simulink model "oven_model"  (R2026a)
settings: Solver=ode15s  StopTime=3600
values from neighbouring files (symbols this model uses):
  A_chimney = pi * D_chimney^2 / 4    (= 0.00785398163397)    [oven_parameters.m]    (also in oven_parameters_V1.m)
  A_floor = W_floor * L_floor    (= 0.3239)    [oven_parameters.m]    (also in oven_parameters_V1.m)
  A_pizza = pi * D_pizza^2 / 4    (= 0.0804247719319)    [oven_parameters.m]    (also in oven_parameters_V1.m)
  A_rad_roof_floor = A_floor    (= 0.3239)    [oven_parameters.m]    (also in oven_parameters_V1.m)
  A_rad_roof_pizza = A_pizza    (= 0.0804247719319)    [oven_parameters.m]    (also in oven_parameters_V1.m)
  A_roof = A_floor    (= 0.3239)    [oven_parameters.m]    (also in oven_parameters_V1.m)
  C_floor = m_floor * cp_floor    (= 7579.26)    [oven_parameters.m]    (also in oven_parameters_V1.m)
  C_gas = m_gas * cp_gas    (= 136.917)    [oven_parameters.m]    (also in oven_parameters_V1.m)
  C_pizza = m_pizza * cp_pizza    (= 625)    [oven_parameters.m]    (also in oven_parameters_V1.m)
  C_roof = m_roof * cp_roof    (= 2526.42)    [oven_parameters.m]    (also in oven_parameters_V1.m)
  Cd_chimney = 0.65    [oven_parameters.m]    (also in oven_parameters_V1.m)
  cp_gas = 1100    [oven_parameters.m]    (also in oven_parameters_V1.m)
  epsilon_pizza = 0.9    [oven_parameters.m]    (also in oven_parameters_V1.m)
  epsilon_roof = 0.8    [oven_parameters.m]    (also in oven_parameters_V1.m)
  g = oven_geometry(p)    [build_oven_simulink.m]    (also in oven_parameters.m = 9.81; oven_parameters_V1.m = 9.81; oven_refresh_model.m; run_oven_study.m = s.results{1}.g)
  H_chimney = 0.50    (= 0.5)    [oven_parameters.m]    (also in oven_parameters_V1.m)
  h_floor_pizza = 150    [oven_parameters.m]    (also in oven_parameters_V1.m)
  h_gas_floor = 20    [oven_parameters.m]    (also in oven_parameters_V1.m)
  h_gas_pizza = 10    [oven_parameters.m]    (also in oven_parameters_V1.m)
  h_gas_roof = 15    [oven_parameters.m]    (also in oven_parameters_V1.m)
  k_evap = 1e-5    (= 1e-05)    [oven_parameters.m]    (also in oven_parameters_V1.m)
  K_floor = 8    [oven_parameters.m]    (also in oven_parameters_V1.m)
  K_roof = 5    [oven_parameters.m]    (also in oven_parameters_V1.m)
  L_vap = 2.26e6    (= 2260000)    [oven_parameters.m]    (also in oven_parameters_V1.m)
  m_water_0 = water_fraction * m_pizza    (= 0.15)    [oven_parameters.m]    (also in oven_parameters_V1.m)
  P_ambient = 101325    [oven_parameters.m]    (also in oven_parameters_V1.m)
  Q_comb = mdot_wood * LHV_wood * eta_comb    (= 13755)    [oven_parameters.m]    (also in oven_parameters_V1.m = 5250)
  R_air = 287    [oven_parameters.m]    (also in oven_parameters_V1.m)
  rho_ambient = P_ambient / (R_air * T_ambient)    (= 1.184131412)    [oven_parameters.m]    (also in oven_parameters_V1.m)
  sigma = 5.670374419e-8    (= 5.670374419e-08)    [oven_parameters.m]    (also in oven_parameters_V1.m)
  T_ambient = 25 + 273.15    (= 298.15)    [oven_parameters.m]    (also in oven_parameters_V1.m)
  T_evap = 373.15    [oven_parameters.m]    (also in oven_parameters_V1.m)
  T_floor_0 = T_ambient    (= 298.15)    [oven_parameters.m]    (also in oven_parameters_V1.m)
  T_gas_0 = T_ambient    (= 298.15)    [oven_parameters.m]    (also in oven_parameters_V1.m)
  T_pizza_0 = T_ambient    (= 298.15)    [oven_parameters.m]    (also in oven_parameters_V1.m)
  T_roof_0 = T_ambient    (= 298.15)    [oven_parameters.m]    (also in oven_parameters_V1.m)
settings Model: Creator=samue  LastModifiedBy=samue

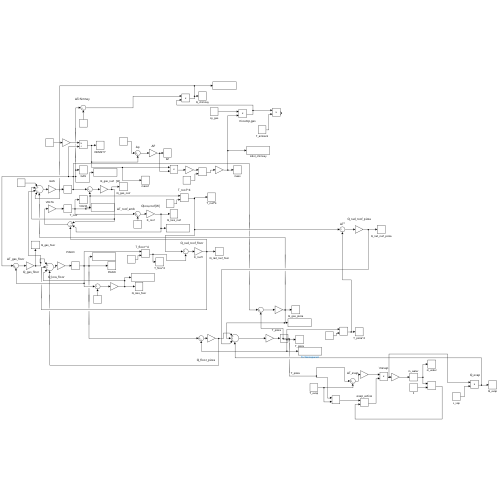
[thumbnail: Simulink's stored preview of the top-level diagram]
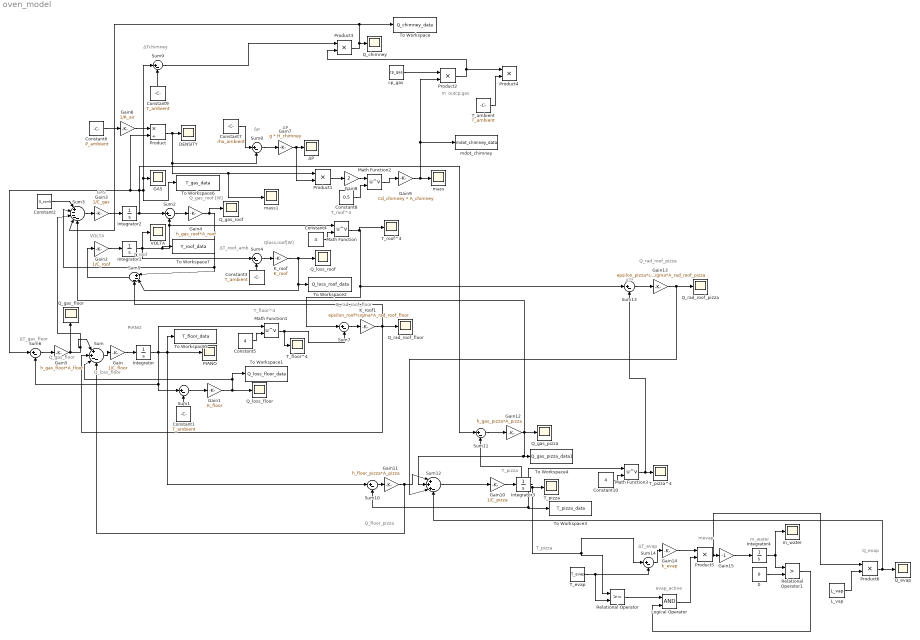
== system oven_model ==
  note: Q_evap
  note: evap_active
  note: ˙mevap​
  note: ΔT_evap
  note: T_pizza
  note: m_water
  note: Q_rad_roof_pizza
  note: ΔT⁴
  note: Q_floor_pizza
  note: T_pizza
  note: ΔTchimney​
  note: m˙out​cp,gas​
  note: ΔP
  note: Δρ
  note: Q_rad_roof_floor
  note: Q_loss_floor
  note: Q_gas_floor
  note: T_floor^4
  note: T_roof^4
  note: ΔT_gas_floor
  note: Qloss,roof​[W]
  note: ΔT_roof_amb
  note: T_roof
  note: Q_gas_roof [W]
  note: GAS
  note: VOLTA
  note: PIANO
  0 : Constant  Value=0
  Constant1 : Constant  Value=T_ambient
  Constant10 : Constant  Value=4
  Constant2 : Constant  Value=Q_comb
  Constant3 : Constant  Value=T_ambient
  Constant4 : Constant  Value=4
  Constant5 : Constant  Value=4
  Constant6 : Constant  Value=P_ambient
  Constant7 : Constant  Value=rho_ambient
  Constant8 : Constant  Value=0.5
  Constant9 : Constant  Value=T_ambient
  DENSITY : Scope
      settings: ActiveDisplayYMinimum=-0.56030182156001862  ActiveDisplayYMaximum=1.4111972218569013  DataLoggingVariableName=ScopeData3
  GAS : Scope
      settings: ActiveDisplayYMinimum=258.3429659927196  ActiveDisplayYMaximum=656.41330606552378
  Gain : Gain  Gain=1/C_floor
  Gain1 : Gain  Gain=K_floor
  Gain10 : Gain  Gain=1/C_pizza
  Gain11 : Gain  Gain=h_floor_pizza*A_pizza
  Gain12 : Gain  Gain=h_gas_pizza*A_pizza
  Gain13 : Gain  Gain=epsilon_pizza*sigma*A_rad_roof_pizza
  Gain14 : Gain  Gain=k_evap
  Gain15 : Gain  Gain=-1
  Gain2 : Gain  Gain=1/C_roof
  Gain3 : Gain  Gain=1/C_gas
  Gain4 : Gain  Gain=h_gas_roof*A_roof
  Gain5 : Gain  Gain=h_gas_floor*A_floor
  Gain6 : Gain  Gain=1/R_air
  Gain7 : Gain  Gain=g * H_chimney
  Gain8 : Gain  Gain=2
  Gain9 : Gain  Gain=Cd_chimney * A_chimney
  Integrator : Integrator  InitialCondition=T_floor_0
  Integrator1 : Integrator  InitialCondition=T_roof_0
  Integrator2 : Integrator  InitialCondition=T_gas_0
  Integrator3 : Integrator  InitialCondition=T_pizza_0
  Integrator4 : Integrator  InitialCondition=m_water_0
  K_roof : Gain  Gain=K_roof
  K_roof1 : Gain  Gain=epsilon_roof*sigma*A_rad_roof_floor
  L_vap : Constant  Value=L_vap
  Logical Operator : Logic  AllPortsSameDT=off  OutDataTypeStr=boolean
  Math Function{,1..3} (4 alike) : Math  Operator=pow
  PIANO : Scope
      settings: ActiveDisplayYMinimum=235.4778080469699  ActiveDisplayYMaximum=862.19972757727112
  Product : Product  Inputs=*/
  Product{1..4} (4 alike) : Product  Inputs=**
  Product5 : Product
  Product6 : Product
  Q_chimney : Scope
      settings: ActiveDisplayYMinimum=-981.18771548625477  ActiveDisplayYMaximum=8830.6894393762959  DataLoggingVariableName=Q_chimney_data
  Q_evap : Scope
      settings: ActiveDisplayYMinimum=-1268.2904261134306  ActiveDisplayYMaximum=11414.613835020878  DataLoggingVariableName=ScopeData20
  Q_gas_floor : Scope
      settings: ActiveDisplayYMinimum=-568.21387781314047  ActiveDisplayYMaximum=5113.9249003182649  DataLoggingVariableName=ScopeData9
  Q_gas_pizza : Scope
      settings: ActiveDisplayYMinimum=-24.642470577879937  ActiveDisplayYMaximum=221.7822352009195  DataLoggingVariableName=ScopeData16
  Q_gas_roof : Scope
      settings: ActiveDisplayYMinimum=-143.66606417495345  ActiveDisplayYMaximum=1292.9945775745814  DataLoggingVariableName=ScopeData10
  Q_loss_floor : Scope
      settings: ActiveDisplayYMinimum=-501.37753562424086  ActiveDisplayYMaximum=4512.3978206181691  DataLoggingVariableName=ScopeData11
  Q_loss_roof : Scope
      settings: ActiveDisplayYMinimum=-316.41135252661337  ActiveDisplayYMaximum=2847.7021727395208  DataLoggingVariableName=ScopeData15
  Q_rad_roof_floor : Scope
      settings: ActiveDisplayYMinimum=-13.468128699934045  ActiveDisplayYMaximum=121.21315829940644  DataLoggingVariableName=ScopeData12
  Q_rad_roof_pizza : Scope
      settings: ActiveDisplayYMinimum=-15.029157613821152  ActiveDisplayYMaximum=25.426795565679427  DataLoggingVariableName=ScopeData18
  Relational Operator : RelationalOperator  OutDataTypeStr=boolean  RndMeth=Simplest  InputSameDT=off
  Relational Operator1 : RelationalOperator  Operator=>  OutDataTypeStr=boolean  RndMeth=Simplest  InputSameDT=off
  Sum : Sum  Inputs=|++--
  Sum{1..2,4,6..11,13..14} (11 alike) : Sum  Inputs=|+-
  Sum12 : Sum  Inputs=|+++-
  Sum3 : Sum  Inputs=|+----
  Sum5 : Sum  Inputs=|+--
  T_ambient : Constant  Value=T_ambient
  T_evap : Constant  Value=T_evap
  T_floor^4 : Scope
      settings: ActiveDisplayYMinimum=-4.2189360590233528E+10  ActiveDisplayYMaximum=4.5872465094973682E+11  DataLoggingVariableName=ScopeData14
  T_pizza : Scope
      settings: ActiveDisplayYMinimum=232.78079290987318  ActiveDisplayYMaximum=886.47286381114156  DataLoggingVariableName=ScopeData7
  T_pizza^4 : Scope
      settings: ActiveDisplayYMinimum=3.7007260322625837E+9  ActiveDisplayYMaximum=4.57138713472718E+10  DataLoggingVariableName=ScopeData17
  T_roof^4 : Scope
      settings: ActiveDisplayYMinimum=-4.3448055988394592E+10  ActiveDisplayYMaximum=4.7005290953318646E+11  DataLoggingVariableName=ScopeData13
  To Workspace : ToWorkspace  VariableName=Q_chimney_data  SaveFormat=Timeseries  SampleTime=-1
  To Workspace1 : ToWorkspace  VariableName=Q_loss_floor_data  SaveFormat=Timeseries  SampleTime=-1
  To Workspace2 : ToWorkspace  VariableName=Q_loss_roof_data  SaveFormat=Timeseries  SampleTime=-1
  To Workspace3 : ToWorkspace  VariableName=T_pizza_data  SaveFormat=Timeseries  SampleTime=-1
  To Workspace4 : ToWorkspace  VariableName=Q_gas_pizza_data1  SaveFormat=Timeseries  SampleTime=-1
  To Workspace5 : ToWorkspace  VariableName=T_floor_data  SaveFormat=Timeseries  SampleTime=-1
  To Workspace6 : ToWorkspace  VariableName=T_gas_data  SaveFormat=Timeseries  SampleTime=-1
  To Workspace7 : ToWorkspace  VariableName=T_roof_data  SaveFormat=Timeseries  SampleTime=-1
  VOLTA : Scope
      settings: ActiveDisplayYMinimum=279.60884636981444  ActiveDisplayYMaximum=465.02038267167012  DataLoggingVariableName=ScopeData2
  cp_gas : Constant  Value=cp_gas
  m_water : Scope
      settings: ActiveDisplayYMinimum=-0.018750000000146448  ActiveDisplayYMaximum=0.16875000000001625  DataLoggingVariableName=ScopeData19
  mass : Scope
      settings: ActiveDisplayYMinimum=-0.0013867918679163283  ActiveDisplayYMaximum=0.011024464304673912  DataLoggingVariableName=ScopeData5
  mass1 : Scope
      settings: ActiveDisplayYMinimum=0.1941441920714547  ActiveDisplayYMaximum=1.294129991992079  DataLoggingVariableName=ScopeData6
  mdot_chimney : ToWorkspace  VariableName=mdot_chimney_data  SaveFormat=Timeseries  SampleTime=-1
  ΔP : Scope
      settings: ActiveDisplayYMinimum=-0.53954303486106625  ActiveDisplayYMaximum=4.855887313749597  DataLoggingVariableName=ScopeData4
  wires:
  Sum1/1 -> Gain1/1
  Integrator/1 -> Math Function1/1, To Workspace5/1, PIANO/1, Sum10/1, Sum6/2, Sum1/1
  Constant1/1 -> Sum1/2
  Gain/1 -> Integrator/1
  Gain1/1 -> To Workspace1/1, Sum/3, Q_loss_floor/1
  Gain2/1 -> Integrator1/1
  Gain3/1 -> Integrator2/1
  Integrator2/1 -> Sum2/1, Sum11/1, Sum9/1, GAS/1, To Workspace6/1, Product/2, Sum6/1
  Integrator1/1 -> To Workspace7/1, Sum2/2, Math Function/1, Sum4/1, VOLTA/1
  Sum2/1 -> Gain4/1
  Gain4/1 -> Q_gas_roof/1, Sum5/1, Sum3/2
  Sum3/1 -> Gain3/1
  Constant2/1 -> Sum3/1
  Constant3/1 -> Sum4/2
  Sum4/1 -> K_roof/1
  K_roof/1 -> Q_loss_roof/1, Sum5/2, To Workspace2/1
  Sum5/1 -> Gain2/1
  Sum6/1 -> Gain5/1
  Gain5/1 -> Sum3/3, Sum/1, Q_gas_floor/1
  Sum/1 -> Gain/1
  Constant4/1 -> Math Function/2
  Constant5/1 -> Math Function1/2
  Math Function/1 -> T_roof^4/1, Sum13/1, Sum7/1
  Math Function1/1 -> T_floor^4/1, Sum7/2
  Sum7/1 -> K_roof1/1
  K_roof1/1 -> Q_rad_roof_floor/1, Sum5/3, Sum/2
  Gain6/1 -> Product/1
  Constant6/1 -> Gain6/1
  Product/1 -> mass1/1, Product1/1, Sum8/2, DENSITY/1
  Constant7/1 -> Sum8/1
  Sum8/1 -> Gain7/1
  Gain7/1 -> Product1/2, ΔP/1
  Product1/1 -> Gain8/1
  Gain8/1 -> Math Function2/1
  Math Function2/1 -> Gain9/1
  Gain9/1 -> mdot_chimney/1, Product2/2, mass/1
  Constant8/1 -> Math Function2/2
  Constant9/1 -> Sum9/2
  cp_gas/1 -> Product2/1
  Product2/1 -> Product4/1, Product3/2
  Sum9/1 -> Product3/1
  Product3/1 -> Q_chimney/1, To Workspace/1, Sum3/4
  T_ambient/1 -> Product4/2
  Gain10/1 -> Integrator3/1
  Integrator3/1 -> Math Function3/1, Sum14/1, Relational Operator/1, T_pizza/1, To Workspace3/1, Sum10/2, Sum11/2
  Sum10/1 -> Gain11/1
  Gain11/1 -> Sum/4, Sum12/1
  Sum11/1 -> Gain12/1
  Gain12/1 -> Sum3/5, Sum12/2, To Workspace4/1, Q_gas_pizza/1
  Sum12/1 -> Gain10/1
  Constant10/1 -> Math Function3/2
  Math Function3/1 -> Sum13/2, T_pizza^4/1
  Sum13/1 -> Gain13/1
  Gain13/1 -> Q_rad_roof_pizza/1, Sum12/3
  T_evap/1 -> Sum14/2, Relational Operator/2
  Sum14/1 -> Gain14/1
  Gain14/1 -> Product5/1
  Product5/1 -> Product6/1, Gain15/1
  Gain15/1 -> Integrator4/1
  Integrator4/1 -> m_water/1, Relational Operator1/1
  0/1 -> Relational Operator1/2
  Relational Operator/1 -> Logical Operator/1
  Relational Operator1/1 -> Logical Operator/2
  Logical Operator/1 -> Product5/2
  L_vap/1 -> Product6/2
  Product6/1 -> Sum12/4, Q_evap/1
